simulink model "multinode_simulink"  (R2018b)
settings: Solver=ode15s  StartTime=0.0  StopTime=10  FixedStep=0.001  MaxStep=0.1  RelTol=1e-3  AbsTol=1e-3
undefined symbols (not defined in the file or in its folder): elevon_max_deflection, kd_aileron, kd_elev, Kd_z, ki_aileron, ki_elev, kp_aileron, kp_elev, Kp_z, N, P_cs_mat, set_roll, t_aileron, t_elev, wce_z, winc_vel_up_lims, X0
settings Model: Creator=Ayaz  LastModifiedBy=Ayaz

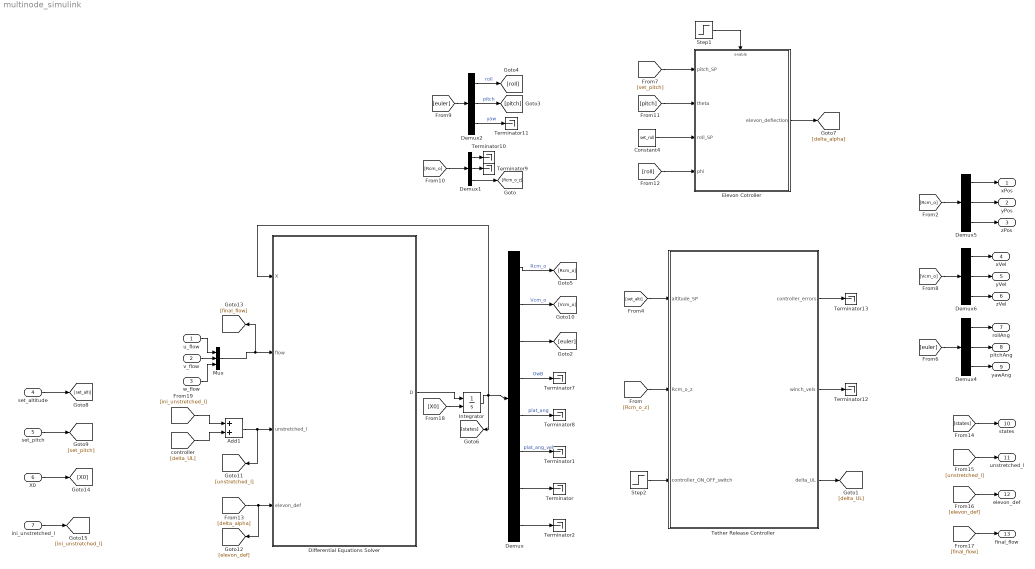
== system multinode_simulink ==
  u_flow : Inport
  v_flow : Inport  Port=2
  w_flow : Inport  Port=3
  set_altitude : Inport  Port=4
  set_pitch : Inport  Port=5
  X0 : Inport  Port=6  PortDimensions=14+18*N
  "ini_unstretched_l " : Inport  Port=7  PortDimensions=3
  Add1 : Sum
  Constant4 : Constant  Value=set_roll
  Demux : Demux  Outputs=[3,3,3,3,1,1,-1,-1]
  Demux{1..2,4..6} (5 alike) : Demux  Outputs=3
  Differential Equations Solver : MATLAB Function  TreatAsAtomicUnit=on
  Elevon Cotroller : Subsystem
  Integrator : Integrator  InitialConditionSource=external  InitialCondition=X0
  Mux : Mux  Inputs=3
  Step1 : Step  Time=0  SampleTime=0
  Step2 : Step  Time=0  SampleTime=0
  Terminator{,1..2,7..13} (10 alike) : Terminator
  Tether Release Controller : Subsystem
  xPos : Outport
  yPos : Outport  Port=2
  zPos : Outport  Port=3
  xVel : Outport  Port=4
  yVel : Outport  Port=5
  zVel : Outport  Port=6
  rollAng : Outport  Port=7
  pitchAng : Outport  Port=8
  yawAng : Outport  Port=9
  states : Outport  Port=10
  unstretched_l : Outport  Port=11
  elevon_def : Outport  Port=12
  final_flow : Outport  Port=13
  wires:
  Differential Equations Solver/1(D) -> Integrator/1
  Integrator/1 -> Differential Equations Solver/1(X), [states], Demux/1
  Demux/1 -> [Rcm_o]  "Rcm_o"
  Demux/2 -> [Vcm_o]  "Vcm_o"
  Demux/3 -> [euler]
  Demux/4 -> Terminator7/1  "OwB"
  Demux/5 -> Terminator8/1  "plat_ang"
  [ini_unstretched_l] -> Add1/1
  Add1/1 -> [unstretched_l], Differential Equations Solver/3(unstretched_l)
  [delta_UL] -> Add1/2
  [Rcm_o_z] -> Tether Release Controller/2(Rcm_o_z)
  Tether Release Controller/1(controller_errors) -> Terminator13/1
  Tether Release Controller/2(winch_vels) -> Terminator12/1
  Tether Release Controller/3(delta_UL) -> [delta_UL]
  [set_pitch] -> Elevon Cotroller/1(pitch_SP)
  [pitch] -> Elevon Cotroller/2(theta)
  Constant4/1 -> Elevon Cotroller/3(roll_SP)
  [roll] -> Elevon Cotroller/4(phi)
  Elevon Cotroller/1(elevon_deflection) -> [delta_alpha]
  [delta_alpha] -> [elevon_def], Differential Equations Solver/4(elevon_def)
  Step1/1 -> Elevon Cotroller/Enable
  Step2/1 -> Tether Release Controller/3(controller_ON_OFF_switch)
  [set_alti] -> Tether Release Controller/1(altitude_SP)
  [euler] -> Demux4/1
  Demux/8 -> Terminator2/1
  Demux/7 -> Terminator/1
  Demux/6 -> Terminator1/1  "plat_ang_vel"
  [Rcm_o] -> Demux5/1
  [Vcm_o] -> Demux6/1
  Demux5/1 -> xPos/1
  Demux5/3 -> zPos/1
  Demux5/2 -> yPos/1
  Demux6/1 -> xVel/1
  Demux6/2 -> yVel/1
  Demux6/3 -> zVel/1
  Demux4/1 -> rollAng/1
  Demux4/2 -> pitchAng/1
  Demux4/3 -> yawAng/1
  Demux2/1 -> [roll]  "roll"
  Demux2/3 -> Terminator11/1  "yaw"
  [euler] -> Demux2/1
  Demux2/2 -> [pitch]  "pitch"
  Demux1/1 -> Terminator10/1
  Demux1/2 -> Terminator9/1
  Demux1/3 -> [Rcm_o_z]
  [Rcm_o] -> Demux1/1
  [states] -> states/1
  [unstretched_l] -> unstretched_l/1
  [elevon_def] -> elevon_def/1
  [final_flow] -> final_flow/1
  set_altitude/1 -> [set_alti]
  set_pitch/1 -> [set_pitch]
  [X0] -> Integrator/2
  X0/1 -> [X0]
  "ini_unstretched_l "/1 -> [ini_unstretched_l]
  v_flow/1 -> Mux/2
  u_flow/1 -> Mux/1
  w_flow/1 -> Mux/3
  Mux/1 -> [final_flow], Differential Equations Solver/2(flow)

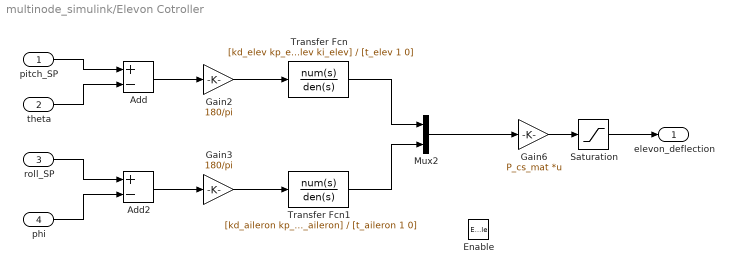
== system multinode_simulink/Elevon Cotroller ==
  pitch_SP : Inport
  theta : Inport  Port=2
  roll_SP : Inport  Port=3
  phi : Inport  Port=4
  Enable : EnablePort
  Add : Sum  Inputs=+-
  Add2 : Sum  Inputs=+-
  Gain2 : Gain  Gain=180/pi
  Gain3 : Gain  Gain=180/pi
  Gain6 : Gain  Gain=P_cs_mat  Multiplication=Matrix(K*u)
  Mux2 : Mux  Inputs=2
  Saturation : Saturate  UpperLimit=elevon_max_deflection  LowerLimit=-elevon_max_deflection
  Transfer Fcn : TransferFcn  Numerator=[kd_elev kp_elev ki_elev]  Denominator=[t_elev 1 0]
  Transfer Fcn1 : TransferFcn  Numerator=[kd_aileron kp_aileron ki_aileron]  Denominator=[t_aileron 1 0]
  elevon_deflection : Outport
  wires:
  Add/1 -> Gain2/1
  Gain3/1 -> Transfer Fcn1/1
  Gain2/1 -> Transfer Fcn/1
  roll_SP/1 -> Add2/1
  Gain6/1 -> Saturation/1
  theta/1 -> Add/2
  pitch_SP/1 -> Add/1
  Add2/1 -> Gain3/1
  Saturation/1 -> elevon_deflection/1
  phi/1 -> Add2/2
  Transfer Fcn/1 -> Mux2/1
  Transfer Fcn1/1 -> Mux2/2
  Mux2/1 -> Gain6/1

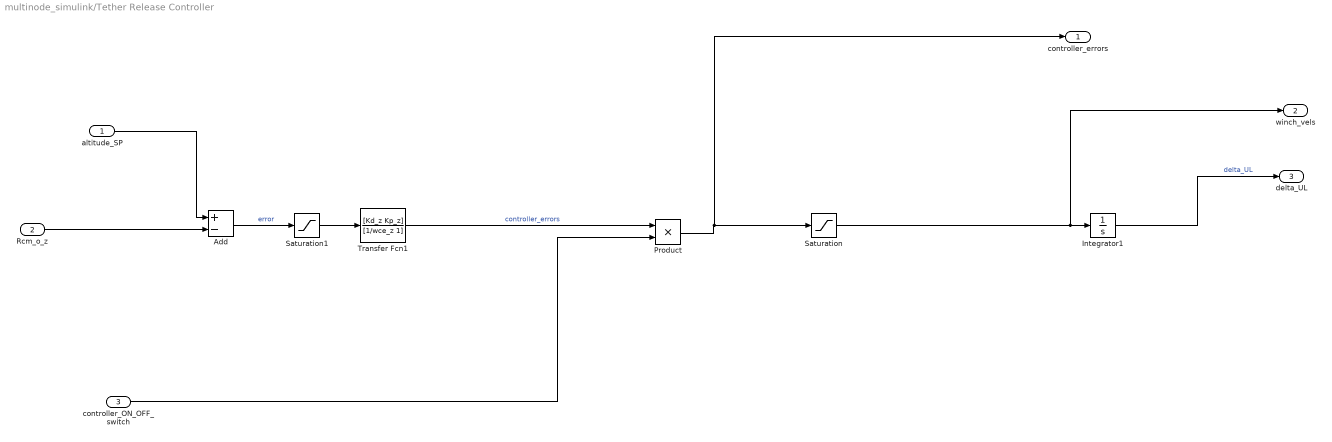
== system multinode_simulink/Tether Release Controller ==
  altitude_SP : Inport
  Rcm_o_z : Inport  Port=2
  controller_ON_OFF_switch : Inport  Port=3
  Add : Sum  Inputs=+-
  Integrator1 : Integrator
  Product : Product
  Saturation : Saturate  UpperLimit=winc_vel_up_lims  LowerLimit=-winc_vel_up_lims
  Saturation1 : Saturate  UpperLimit=5  LowerLimit=-5
  Transfer Fcn1 : TransferFcn  Numerator=[Kd_z Kp_z]  Denominator=[1/wce_z 1]
  controller_errors : Outport
  winch_vels : Outport  Port=2
  delta_UL : Outport  Port=3
  wires:
  Integrator1/1 -> delta_UL/1  "delta_UL"
  Add/1 -> Saturation1/1  "error"
  altitude_SP/1 -> Add/1
  Rcm_o_z/1 -> Add/2
  Saturation1/1 -> Transfer Fcn1/1
  Product/1 -> Saturation/1, controller_errors/1
  Saturation/1 -> winch_vels/1, Integrator1/1
  Transfer Fcn1/1 -> Product/1  "controller_errors"
  controller_ON_OFF_switch/1 -> Product/2

== matlab function multinode_simulink/Differential Equations Solver ==
  data: X input; D output; flow input; unstretched_l input; elevon_def input; sim_param parameter
function D = multimode_ode(X,flow,unstretched_l,elevon_def,sim_param)

D = zeros(size(X));

% loader = load('sim_param.mat');
% 
% sim_param = loader.sim_param;

%% number of nodes
N = sim_param.N;

% extract other values
mass = sim_param.geom_param.mass;
MI = sim_param.geom_param.MI;

P_Izz = sim_param.platform_param.platform_Izz;
cp = sim_param.platform_param.platform_damping;

R2n_cm = sim_param.tether_imp_nodes.R2n_cm;

R21_g = sim_param.tether_imp_nodes.R21_g;


%% constants
m = mass;
Ixx = MI(1,1);
Iyy = MI(2,2);
Izz = MI(3,3);

m_added = sim_param.geom_param.m_added;
Izz_added = sim_param.geom_param.Izz_added;

%% extract values from state space
% lifting body values
Rcm_o = X(1:3,1);
O_Vcm_o = X(4:6,1);

euler_ang = X(7:9,1);
ph = euler_ang(1);
th = euler_ang(2);
ps = euler_ang(3);

% rotations
[oCb,bCo] = rotation_sequence(euler_ang);

OwB = X(10:12,1);
wx = OwB(1);
wy = OwB(2);
wz = OwB(3);

psi_p = X(13,1);
platform_ang_vel = X(14,1);

pCo = [cos(psi_p) sin(psi_p) 0; -sin(psi_p) cos(psi_p) 0; 0 0 1];
oCp = pCo';


% tether position and velocity components
R2i_o = X(15:(14 + 3*N),1);
O_V2i_o = X((15 + 3*N):(14 + 6*N),1);

%%  center of mass first derivatives
D(1:3,1) = O_Vcm_o;
D(7,1) = wx + sin(ph)*tan(th)*wy + cos(ph)*tan(th)*wz;
D(8,1) = cos(ph)*wy - sin(ph)*wz;
D(9,1) = sec(th)*sin(ph)*wy + cos(ph)*sec(th)*wz;

%% platofrm angle first derivates
D(13,1) = platform_ang_vel;
OwP = [0;0;platform_ang_vel];

%% changing first node first deivative
O_V2i_o(1:3,1) = oCp*(cross(OwP,R21_g));

%% changing last node first deivative
O_V2i_o((end-2):end,1)=  O_Vcm_o + oCb*(cross(OwB,R2n_cm));

%% tether nodes first derivatives
D(15:(14 + 3*N),1) = O_V2i_o;


%% EXTERNAL FORCES AND TORQUES
op = multinode_F_and_T_external(sim_param,flow,unstretched_l,elevon_def,Rcm_o,R2i_o,...
    O_Vcm_o,O_V2i_o,OwB,euler_ang,psi_p);

O_F_ext = op.O_F_ext;
B_T_ext = op.B_T_ext;
sum_2_f = op.sum_2_f;
T_o_ext = op.T_o_ext;

Tx = B_T_ext(1);
Ty = B_T_ext(2);
Tz = B_T_ext(3);

% mass at each node
tether_masses = op.tether_masses;

m2i = tether_masses/N;

%% center of mass second derivatives
% added mass
mass_matrix = [1/(m+m_added(1)) 0 0;0 1/(m+m_added(2)) 0;0 0 1/(m+m_added(3))];

D(4:6,1) = oCb*(mass_matrix*(bCo*O_F_ext));
D(10,1) = (1/Ixx)*(Tx + (Iyy - Izz)*wy*wz);
D(11,1) = (1/Iyy)*(Ty + (Izz - Ixx)*wx*wz);
D(12,1) = (1/(Izz+Izz_added))*(Tz + (Ixx - Iyy)*wx*wy);

OaB = D(10:12,1);

%% platform angle second derivative
D(14,1) = (T_o_ext/P_Izz) - cp*platform_ang_vel;
OaP = [0;0;D(14,1)];

%% tether nodes 2nd derivatives
for i = 1:N
    if i == 1
        D((14 + 3*N + 3*i - 2):(14 + 3*N + 3*i),1) = oCp*( cross(OaP,R21_g) +  cross(OwP,(cross(OwP,R21_g))) );
        
    elseif i>1 && i<N
        D((14 + 3*N + 3*i - 2):(14 + 3*N + 3*i),1) = (1/m2i)*sum_2_f(:,i);
        
    elseif i == N
        D((14 + 3*N + 3*i - 2):(14 + 3*N + 3*i),1) =  D(4:6,1) + ...
            oCb*( cross(OaB,R2n_cm) +  cross(OwB,(cross(OwB,R2n_cm))) ) ;
    end
end

end
